simulink model "TestPWMGenerator"  (R2020b)
settings: Solver=FixedStepAuto  StartTime=0.0  StopTime=250  RelTol=1e-3  EnableMultiTasking=on
model workspace (MAT data in the model file):
  T = 1
undefined symbols (not defined in the file): DiscIntNeverNeededParam
libraries: bbblueBasicLib x2, simulink x1
settings Model: ExtModeTrigDuration=100  Creator=Zein  LastModifiedBy=Zein
settings SolverCC: PositivePriorityOrder=on
settings OptimizationCC: EnhancedBackFolding=on  PassReuseOutputArgsAs=Individual arguments  ZeroExternalMemoryAtStartup=off  ZeroInternalMemoryAtStartup=off  MaxStackSize=64  OptimizeBlockOrder=speed  DifferentSizesBufferReuse=on  OptimizationCustomize=off  EfficientTunableParamExpr=on
settings DebuggingCC: ParameterTunabilityLossMsg=error
settings HardwareCC: ProdBitPerPointer=32  ProdBitPerSizeT=32  ProdBitPerPtrDiffT=32  ProdLargestAtomicInteger=Long  ProdLargestAtomicFloat=Double  ProdWordSize=32  ProdHWDeviceType=ARM Compatible->ARM Cortex
settings SFSimCC: MATLABDynamicMemAlloc=off
settings RTWCC: Description=Embedded Coder  SystemTargetFile=ert.tlc  HardwareBoard=BeagleBone Blue  TLCOptions="-aInlineSetEventsForThisBaseRateFcn=TLC_FALSE -aSuppressMultiTaskScheduler=TLC_FALSE  -aRateBasedStepFcn=0"  TemplateMakefile=ert_default_tmf  Toolchain=GNU GCC BeagleBone Blue
settings CodeAppCC: ForceParamTrailComments=on  IgnoreCustomStorageClasses=off  OperatorAnnotations=on  SimulinkDataObjDesc=on  SFDataObjDesc=on  InsertBlockDesc=on
settings ERTTargetCC: MatFileLogging=on  SupportVariableSizeSignals=on

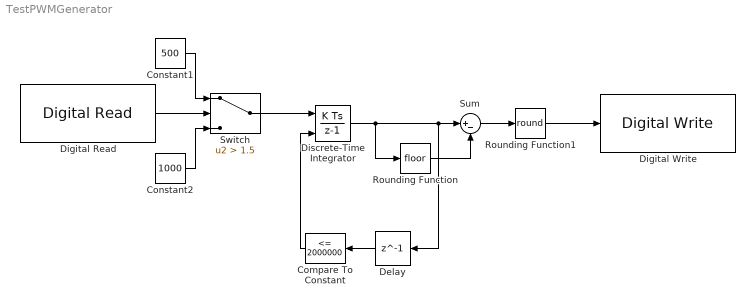
== system TestPWMGenerator ==
  Compare To Constant : simulink/Logic and Bit Operations/Compare To Constant  relop=<=  const=2000000  OutDataTypeStr=boolean
  Constant1 : Constant  Value=500
  Constant2 : Constant  Value=1000
  Delay : Delay  DelayLength=1
  Digital Read : bbblueBasicLib/Digital Read  Pin=49  Direction=input  GPIOSelect=GPIO3_2  SampleTime=-1
      settings: SourceProductBaseCode=SC_BEAGLEBONE_BLUE
  Digital Write : bbblueBasicLib/Digital Write  GPIOSelect=GPIO3_1  Pin=49  Direction=output
      settings: SourceProductBaseCode=SC_BEAGLEBONE_BLUE
  Discrete-Time Integrator : DiscreteIntegrator  ExternalReset=rising  SampleTime=1/5000  ICPrevOutput=DiscIntNeverNeededParam  ICPrevScaledInput=DiscIntNeverNeededParam
  Rounding Function : Rounding
  Rounding Function1 : Rounding  Operator=round
  Sum : Sum  Inputs=|+-
  Switch : Switch  Criteria=u2 > Threshold  Threshold=1.5
  wires:
  Discrete-Time Integrator/1 -> Delay/1, Sum/1, Rounding Function/1
  Rounding Function/1 -> Sum/2
  Sum/1 -> Rounding Function1/1
  Rounding Function1/1 -> Digital Write/1
  Digital Read/1 -> Switch/2
  Switch/1 -> Discrete-Time Integrator/1
  Constant1/1 -> Switch/1
  Constant2/1 -> Switch/3
  Compare To Constant/1 -> Discrete-Time Integrator/2
  Delay/1 -> Compare To Constant/1
